simulink model "rc_circuit"  (R2026a)
settings: Solver=VariableStepAuto  StopTime=86400
undefined symbols (not defined in the file or in its folder): C, R
settings Model: Creator=frenc  LastModifiedBy=frenc

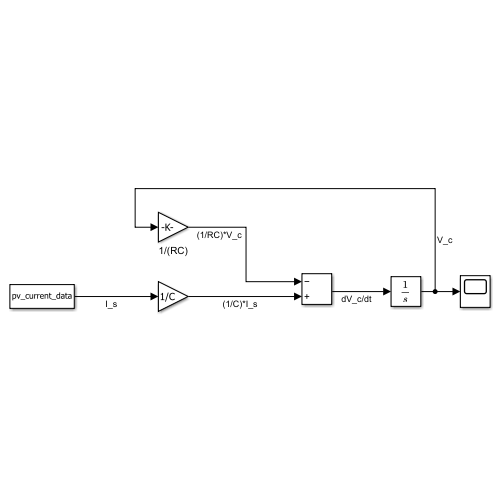
[thumbnail: Simulink's stored preview of the top-level diagram]
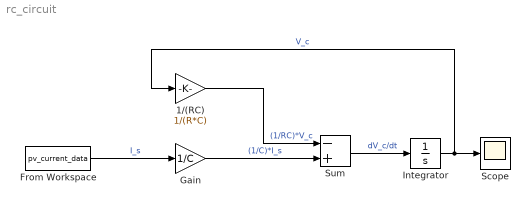
== system rc_circuit ==
  1/(RC) : Gain  Gain=1/(R*C)
  From Workspace : FromWorkspace  VariableName=pv_current_data  SampleTime=-1
  Gain : Gain  Gain=1/C
  Integrator : Integrator
  Scope : Scope
      settings: ActiveDisplayYMinimum=-2.8231864237448741  ActiveDisplayYMaximum=6.0916752189534584
  Sum : Sum  Inputs=-+
  wires:
  From Workspace/1 -> Gain/1  "I_s"
  Gain/1 -> Sum/2  "(1/C)*I_s"
  Sum/1 -> Integrator/1  "dV_c/dt"
  1/(RC)/1 -> Sum/1  "(1/RC)*V_c"
  Integrator/1 -> 1/(RC)/1, Scope/1  "V_c"
